simulink model "robot_model_no_yaw"  (R2024b)
settings: Solver=VariableStepAuto  StartTime=0.0  StopTime=10.0  RelTol=1e-3
values from neighbouring files (symbols this model uses):
  g = 9.81    [robot.m]    (also in robot_cascade.m; robot_linear.m; robot_lqr.m)
  Jm = J - Jp    (= -0.00204667)    [robot.m]
  Jp = m*l^2    (= 0.002112)    [robot.m]    (also in robot_cascade.m = 6.533e-05; robot_linear.m = 6.533e-05; robot_lqr.m = 6.533e-05)
  Jp_delta = 9.0372e-5    (= 9.0372e-05)    [robot.m]
  Jw = 1/2*Mw*R^2    (= 4e-07)    [robot.m]    (also in robot_cascade.m = 1e-08; robot_linear.m; robot_lqr.m = 1e-08)
  Km = 0.212207    [robot.m]    (also in robot_cascade.m = 16.1290322581; robot_linear.m; robot_lqr.m)
  l = 0.08    [robot.m]    (also in robot_cascade.m; robot_linear.m)
  l_axel = 0.2359    [robot.m]    (also in robot_cascade.m; robot_linear.m; robot_lqr.m)
  M = 1.180    (= 1.18)    [robot.m]    (also in robot_cascade.m; robot_linear.m; robot_lqr.m)
  m = 0.33    [robot.m]    (also in robot_cascade.m; robot_linear.m; robot_lqr.m)
  Mw = 0.0005    [robot.m]    (also in robot_linear.m)
  n = 18.75    [robot.m]    (also in robot_cascade.m; robot_linear.m; robot_lqr.m)
  R = 1    [invgui.m]    (also in robot.m = 0.04; robot_lqr.m = 200)
libraries: dspsrcs4 x2, cstblocks x2, dspsigops x2, slpidlib x2, simulink_extras x1
settings Model: Creator=cosr3  LastModifiedBy=cosr3

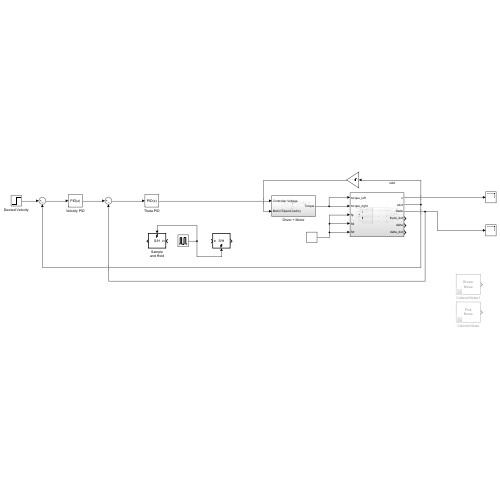
[thumbnail: Simulink's stored preview of the top-level diagram]
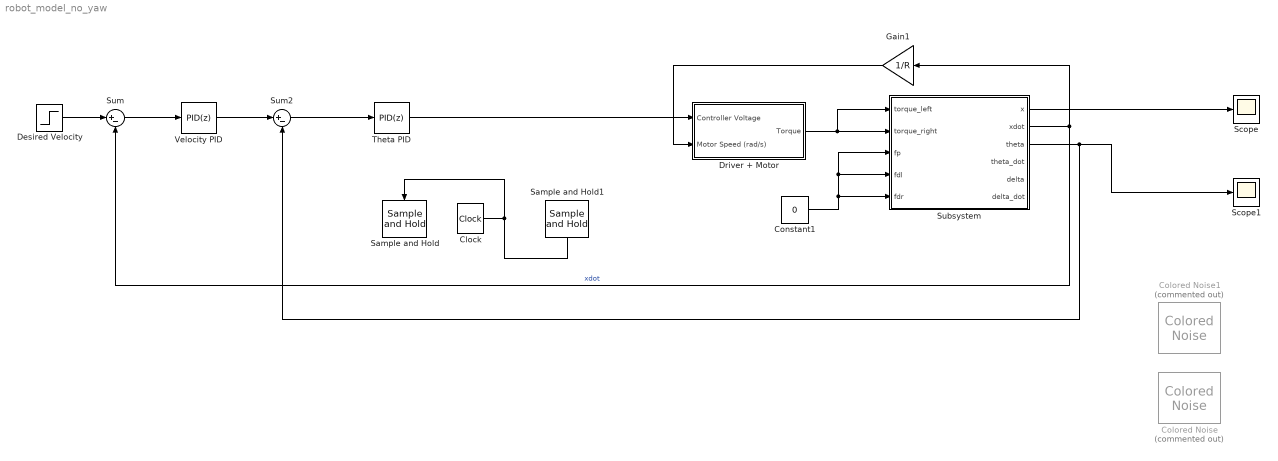
== system robot_model_no_yaw ==
  Clock : simulink_extras/Flip Flops/Clock  period=0.025
  Colored Noise : dspsrcs4/Colored Noise  Commented=on  Color=pink  InverseFrequencyPower=1  BoundedOutput=on  NumChannels=1  OutputDataType=double  SamplesPerFrame=1024  SampleTime=1  RandomStream=mt19937ar with seed  Seed=67  SimulateUsing=Interpreted execution
  Colored Noise1 : dspsrcs4/Colored Noise  Commented=on  Color=brown  InverseFrequencyPower=1  BoundedOutput=on  NumChannels=1  OutputDataType=double  SamplesPerFrame=1024  SampleTime=1  RandomStream=mt19937ar with seed  Seed=67  SimulateUsing=Interpreted execution
  Constant1 : Constant  Value=0
  Desired Velocity : Step  SampleTime=0
  Driver + Motor : Subsystem
  Gain1 : Gain  Gain=1/R
  Sample and Hold : dspsigops/Sample and Hold  trig=Rising edge  initCond=0  latchinput=off
  Sample and Hold1 : dspsigops/Sample and Hold  trig=Rising edge  initCond=0  latchinput=off
  Scope : Scope
  Scope1 : Scope
  Subsystem : Subsystem
  Sum : Sum  Inputs=|+-
  Sum2 : Sum  Inputs=|+-
  Theta PID : slpidlib/PID Controller  Controller=PID  Form=Parallel  TimeDomain=Discrete-time  UseExternalTs=off  SampleTime=0.001  IntegratorMethod=Forward Euler  FilterMethod=Forward Euler  ControllerParametersSource=internal  P=179.074254592637  I=3047.87312037924  UseKiTs=off  D=0.47873796737071  UseExternalDerivativeSource=off  N=3932.92893034675  UseFilter=on  TunerSelectOption=Transfer Function Based (PID Tuner App)  InitialConditionSource=internal  InitialConditionForIntegrator=0  InitialConditionForFilter=0  DifferentiatorICPrevScaledInput=0  ExternalReset=none  TrackingMode=off  Kt=1  LimitOutput=off  SatLimitsSource=internal  UpperSaturationLimit=inf  LowerSaturationLimit=-inf  LinearizeAsGain=off  AntiWindupMode=none  Kb=1  LimitIntegrator=off  UpperIntegratorSaturationLimit=inf  LowerIntegratorSaturationLimit=-inf  POutMin=[]  POutMax=[]  IOutMin=[]  IOutMax=[]  DOutMin=[]  DOutMax=[]  NOutMin=[]  NOutMax=[]  SumOutMin=[]  SumOutMax=[]  SaturationOutMin=[]  SaturationOutMax=[]  PParamMin=[]  PParamMax=[]  IParamMin=[]  IParamMax=[]  DParamMin=[]  DParamMax=[]  NParamMin=[]  NParamMax=[]  KbParamMin=[]  KbParamMax=[]  KtParamMin=[]  KtParamMax=[]  KbOutMin=[]  KbOutMax=[]  KtOutMin=[]  KtOutMax=[]  IntegratorOutMin=[]  IntegratorOutMax=[]  FilterOutMin=[]  FilterOutMax=[]  SumI1OutMin=[]  SumI1OutMax=[]  SumI2OutMin=[]  SumI2OutMax=[]  SumI3OutMin=[]  SumI3OutMax=[]  SumI4OutMin=[]  SumI4OutMax=[]  SumDOutMin=[]  SumDOutMax=[]  DifferentiatorOutMin=[]  DifferentiatorOutMax=[]  FilterDiffOutCoefMin=[]  FilterDiffOutCoefMax=[]  ReciprocalOutMin=[]  ReciprocalOutMax=[]  SumDenOutMin=[]  SumDenOutMax=[]  SumNumOutMin=[]  SumNumOutMax=[]  DivideOutMin=[]  DivideOutMax=[]  UdiffTsProdOutMin=[]  UdiffTsProdOutMax=[]  NTsProdOutMin=[]  NTsProdOutMax=[]  UintegralTsProdOutMin=[]  UintegralTsProdOutMax=[]  UngainTsProdOutMin=[]  UngainTsProdOutMax=[]  ClampingZeroOutDataTypeStr=Inherit: Inherit via back propagation  ClampingZeroOutMin=[]  ClampingZeroOutMax=[]  FilterDenConstantOutDataTypeStr=Inherit: Inherit via back propagation  FilterDenConstantOutMin=[]  FilterDenConstantOutMax=[]  PCopyOutDataTypeStr=Inherit: Inherit via back propagation  PCopyOutMin=[]  PCopyOutMax=[]  NCopyOutDataTypeStr=Inherit: Inherit via back propagation  NCopyOutMin=[]  NCopyOutMax=[]  IntegratorContinuousStateAttributes=''  IntegratorStateMustResolveToSignalObject=off  IntegratorRTWStateStorageClass=Auto  FilterContinuousStateAttributes=''  FilterStateMustResolveToSignalObject=off  FilterRTWStateStorageClass=Auto  ParallelPVariant=InternalParameters  IdealPVariant=Disabled  IVariant=InternalParameters  DVariant=InternalParameters  IntegratorVariant=Discrete  SatVariant=Disabled  AWVariant=Passthrough  PCopyVariant=Disabled  TRVariant=Disabled  FdbkBlocksVariant=Forward  IdealPFdbkVariant=Disabled  SatFdbkVariant=Disabled  DerivativeFilterVariant=ForwardEulerFilter  NVariant=InternalParameters  NCopyVariant=Disabled  FilterICVariant=InternalICsFilter  IntegratorICVariant=InternalICs  ExternalResetVariant=Disabled  TRSumVariant=Passthrough  SumFdbkVariant=Disabled  SumVariant=Sum_PID  TsampFilterVariant=InternalTs  TsampNgainVariant=Passthrough  TsampIntegralVariant=Disabled_SignalSpec  ExternalSaturationOutDataTypeStr=Inherit: Same as second input  DerivativeSourceVariant=ErrorSignal  PreIntVariant=InternalPreInt
      settings: LibrarySourceBlock=simulink/Discrete/Discrete PID Controller
  Velocity PID : slpidlib/PID Controller  Controller=PID  Form=Parallel  TimeDomain=Discrete-time  UseExternalTs=off  SampleTime=0.0005  IntegratorMethod=Forward Euler  FilterMethod=Forward Euler  ControllerParametersSource=internal  P=-3.8153848655145  I=-2.67639168830918  UseKiTs=off  D=0.0967289560038352  UseExternalDerivativeSource=off  N=39.0521382814013  UseFilter=on  TunerSelectOption=Transfer Function Based (PID Tuner App)  InitialConditionSource=internal  InitialConditionForIntegrator=0  InitialConditionForFilter=0  DifferentiatorICPrevScaledInput=0  ExternalReset=none  TrackingMode=off  Kt=1  LimitOutput=off  SatLimitsSource=internal  UpperSaturationLimit=inf  LowerSaturationLimit=-inf  LinearizeAsGain=off  AntiWindupMode=none  Kb=1  LimitIntegrator=off  UpperIntegratorSaturationLimit=inf  LowerIntegratorSaturationLimit=-inf  POutMin=[]  POutMax=[]  IOutMin=[]  IOutMax=[]  DOutMin=[]  DOutMax=[]  NOutMin=[]  NOutMax=[]  SumOutMin=[]  SumOutMax=[]  SaturationOutMin=[]  SaturationOutMax=[]  PParamMin=[]  PParamMax=[]  IParamMin=[]  IParamMax=[]  DParamMin=[]  DParamMax=[]  NParamMin=[]  NParamMax=[]  KbParamMin=[]  KbParamMax=[]  KtParamMin=[]  KtParamMax=[]  KbOutMin=[]  KbOutMax=[]  KtOutMin=[]  KtOutMax=[]  IntegratorOutMin=[]  IntegratorOutMax=[]  FilterOutMin=[]  FilterOutMax=[]  SumI1OutMin=[]  SumI1OutMax=[]  SumI2OutMin=[]  SumI2OutMax=[]  SumI3OutMin=[]  SumI3OutMax=[]  SumI4OutMin=[]  SumI4OutMax=[]  SumDOutMin=[]  SumDOutMax=[]  DifferentiatorOutMin=[]  DifferentiatorOutMax=[]  FilterDiffOutCoefMin=[]  FilterDiffOutCoefMax=[]  ReciprocalOutMin=[]  ReciprocalOutMax=[]  SumDenOutMin=[]  SumDenOutMax=[]  SumNumOutMin=[]  SumNumOutMax=[]  DivideOutMin=[]  DivideOutMax=[]  UdiffTsProdOutMin=[]  UdiffTsProdOutMax=[]  NTsProdOutMin=[]  NTsProdOutMax=[]  UintegralTsProdOutMin=[]  UintegralTsProdOutMax=[]  UngainTsProdOutMin=[]  UngainTsProdOutMax=[]  ClampingZeroOutDataTypeStr=Inherit: Inherit via back propagation  ClampingZeroOutMin=[]  ClampingZeroOutMax=[]  FilterDenConstantOutDataTypeStr=Inherit: Inherit via back propagation  FilterDenConstantOutMin=[]  FilterDenConstantOutMax=[]  PCopyOutDataTypeStr=Inherit: Inherit via back propagation  PCopyOutMin=[]  PCopyOutMax=[]  NCopyOutDataTypeStr=Inherit: Inherit via back propagation  NCopyOutMin=[]  NCopyOutMax=[]  IntegratorContinuousStateAttributes=''  IntegratorStateMustResolveToSignalObject=off  IntegratorRTWStateStorageClass=Auto  FilterContinuousStateAttributes=''  FilterStateMustResolveToSignalObject=off  FilterRTWStateStorageClass=Auto  ParallelPVariant=InternalParameters  IdealPVariant=Disabled  IVariant=InternalParameters  DVariant=InternalParameters  IntegratorVariant=Discrete  SatVariant=Disabled  AWVariant=Passthrough  PCopyVariant=Disabled  TRVariant=Disabled  FdbkBlocksVariant=Forward  IdealPFdbkVariant=Disabled  SatFdbkVariant=Disabled  DerivativeFilterVariant=ForwardEulerFilter  NVariant=InternalParameters  NCopyVariant=Disabled  FilterICVariant=InternalICsFilter  IntegratorICVariant=InternalICs  ExternalResetVariant=Disabled  TRSumVariant=Passthrough  SumFdbkVariant=Disabled  SumVariant=Sum_PID  TsampFilterVariant=InternalTs  TsampNgainVariant=Passthrough  TsampIntegralVariant=Disabled_SignalSpec  ExternalSaturationOutDataTypeStr=Inherit: Same as second input  DerivativeSourceVariant=ErrorSignal  PreIntVariant=InternalPreInt
      settings: LibrarySourceBlock=simulink/Discrete/Discrete PID Controller
  wires:
  Desired Velocity/1 -> Sum/1
  Subsystem/2(xdot) -> Gain1/1, Sum/2  "xdot"
  Sum2/1 -> Theta PID/1
  Subsystem/1(x) -> Scope/1
  Driver + Motor/1(Torque) -> Subsystem/1(torque_left), Subsystem/2(torque_right)
  Gain1/1 -> Driver + Motor/2(Motor Speed (rad/s))
  Constant1/1 -> Subsystem/4(fdl), Subsystem/3(fp), Subsystem/5(fdr)
  Subsystem/3(theta) -> Sum2/2, Scope1/1
  Clock/1 -> Sample and Hold/Trigger, Sample and Hold1/Trigger
  Sum/1 -> Velocity PID/1
  Theta PID/1 -> Driver + Motor/1(Controller Voltage)
  Velocity PID/1 -> Sum2/1

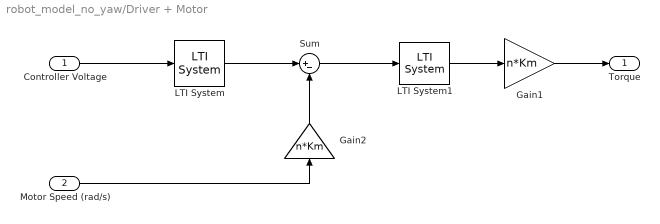
== system robot_model_no_yaw/Driver + Motor ==
  Controller Voltage : Inport
  Motor Speed (rad/s) : Inport  Port=2
  Gain1 : Gain  Gain=n*Km
  Gain2 : Gain  Gain=n*Km
  LTI System : cstblocks/LTI System  sys=Ga  IC=[]  PadeOrder=0
  LTI System1 : cstblocks/LTI System  sys=Ye  IC=[]  PadeOrder=0
  Sum : Sum  Inputs=|+-
  Torque : Outport
  wires:
  Controller Voltage/1 -> LTI System/1
  LTI System1/1 -> Gain1/1
  Gain1/1 -> Torque/1
  LTI System/1 -> Sum/1
  Sum/1 -> LTI System1/1
  Gain2/1 -> Sum/2
  Motor Speed (rad/s)/1 -> Gain2/1

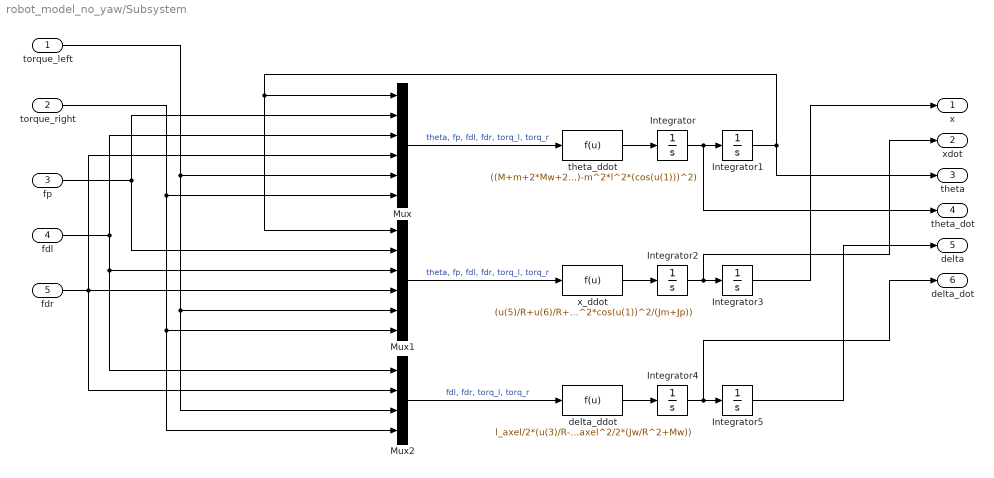
== system robot_model_no_yaw/Subsystem ==
  torque_left : Inport
  torque_right : Inport  Port=2
  fp : Inport  Port=3
  fdl : Inport  Port=4
  fdr : Inport  Port=5
  Integrator : Integrator  ContinuousStateAttributes='theta_dot'
  Integrator1 : Integrator  ContinuousStateAttributes='theta'
  Integrator{2..5} (4 alike) : Integrator
  Mux : Mux  Inputs=6
  Mux1 : Mux  Inputs=6
  Mux2 : Mux
  delta_ddot : Fcn  Expr=l_axel/2*(u(3)/R-u(2)/R+u(1)-u(2))/(Jp_delta+l_axel^2/2*(Jw/R^2+Mw))
  theta_ddot : Fcn  Expr=((M+m+2*Mw+2*Jw/R^2)*(m*g*l*sin(u(1))+u(2)*l*cos(u(1)))-m*l*cos(u(1))*(u(5)/R+u(6)/R+u(2)+u(3)+u(4)))/((Jm+Jp)*(M+m+2*Mw+2*Jw/R^2)-m^2*l^2*(cos(u(1)))^2)
  x_ddot : Fcn  Expr=(u(5)/R+u(6)/R+u(2)+u(3)+u(4)-(m*l*cos(u(1))*(m*g*l*sin(u(1))-u(2)*l*cos(u(1))))/Jm+Jp)/(M+m+2*Mw+2*Jw/R^2-m^2*l^2*cos(u(1))^2/(Jm+Jp))
  x : Outport
  xdot : Outport  Port=2
  theta : Outport  Port=3
  theta_dot : Outport  Port=4
  delta : Outport  Port=5
  delta_dot : Outport  Port=6
  wires:
  theta_ddot/1 -> Integrator/1
  Integrator/1 -> theta_dot/1, Integrator1/1
  Mux/1 -> theta_ddot/1  "theta, fp, fdl, fdr, torq_l, torq_r"
  torque_right/1 -> Mux2/4, Mux1/6, Mux/6
  fp/1 -> Mux/2, Mux1/2
  fdl/1 -> Mux/3, Mux2/1, Mux1/3
  Integrator1/1 -> theta/1, Mux/1, Mux1/1
  torque_left/1 -> Mux2/3, Mux1/5, Mux/5
  Integrator5/1 -> delta/1
  Integrator4/1 -> delta_dot/1, Integrator5/1
  Integrator2/1 -> xdot/1, Integrator3/1
  Integrator3/1 -> x/1
  Mux2/1 -> delta_ddot/1  "fdl, fdr, torq_l, torq_r"
  delta_ddot/1 -> Integrator4/1
  fdr/1 -> Mux2/2, Mux1/4, Mux/4
  x_ddot/1 -> Integrator2/1
  Mux1/1 -> x_ddot/1  "theta, fp, fdl, fdr, torq_l, torq_r"
